simulink model "demoee"  (Simulink 6.3)
settings: Solver=FixedStepDiscrete  StartTime=0.0  StopTime=20  FixedStep=1  RelTol=1e-3
InitFcn:
  | %% DSPBuilder Start
  | alt_dspbuilder_update_model(bdroot)
  | %% DSPBuilder End
libraries: allblocks_alteradspbuilder2 x5
settings Model: LastModifiedBy=delphick
settings OptimizationCC: BlockReduction=off  BooleanDataType=off  InlineInvariantSignals=on
settings DebuggingCC: SolverPrmCheckMsg=none
settings HardwareCC: TargetUnknown=on

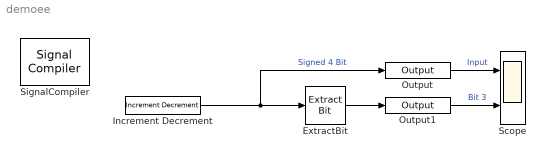
== system demoee ==
  ExtractBit : allblocks_alteradspbuilder2/Extract Bit  BusType=Signed Integer  bwl=4  bwr=0  bitToSelect=3
  Increment Decrement : allblocks_alteradspbuilder2/Increment Decrement  BusType=Signed Integer  bwl=4  bwr=0  SpecifyClock=off  clr_value=0  direction=Increment  phase_selection=1  use_ena=off  use_sclr=off
  Output : allblocks_alteradspbuilder2/Output  iofile=C:\workspace_clean\Documentation\DesignExamples\Tutorials\UnitBlocks\IOBus\ExtractBit\tb_demoee\demoee_Output.capture  BusType=Signed Integer  bwl=4  bwr=0  PORTTYPE=Output
  Output1 : allblocks_alteradspbuilder2/Output  iofile=C:\workspace_clean\Documentation\DesignExamples\Tutorials\UnitBlocks\IOBus\ExtractBit\tb_demoee\demoee_Output1.capture  BusType=Single Bit  bwl=8  bwr=0  PORTTYPE=Output
  Scope : Scope  NumInputPorts=2
      settings: YMin=-9~-1  YMax=8~2
  SignalCompiler : allblocks_alteradspbuilder2/Signal Compiler  DeviceFamily=Stratix IV  DeviceName=AUTO  EnableSignalTap=off  SignalTapDepth=128  UseBoardBlock=off  StpUseDefaultClock=on  StpClock=clock
  wires:
  Increment Decrement/1 -> ExtractBit/1, Output/1  "Signed 4 Bit"
  ExtractBit/1 -> Output1/1
  Output/1 -> Scope/1  "Input"
  Output1/1 -> Scope/2  "Bit 3"
